simulink library "CaffeLibrary"  (Simulink 8.3)
settings: Solver=ode45  StartTime=0.0  StopTime=10.0  RelTol=1e-3
undefined symbols (not defined in the file): c_bias_term_, c_f_max_w, c_f_mean_w, c_f_min_w, c_f_std_w, c_f_type_b, c_f_type_w, c_f_value_w, c_f_variance_norm_w, c_group_, c_kernel_h_, c_kernel_w_, c_num_output_, c_stride_h_, c_stride_w_, EuclideanLoss, loss_weight, misc_, name_, Neuron, p_decay_b, p_decay_w, p_lr_b, p_lr_w, Pooling
settings Model: Creator=twerd  LastModifiedBy=gipadmin

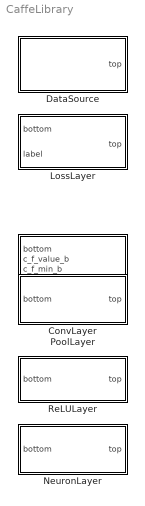
== system CaffeLibrary ==
  ConvLayer : MATLAB Function  TreatAsAtomicUnit=on  mask{title=0, numFilters=24.759999999999998, kernelSize=1.0, stride=0, weightFill=Xavier, weightStd=0, biasFill=0, biasVal=0}
      mask prompts: title "Name"; numFilters "Number of filters"; kernelSize "Kernel size"; weightFill "Type of weights"; weightStd "Std of weights"; biasFill "Type of biases"; biasVal "Bias value"
  DataSource : MATLAB Function  TreatAsAtomicUnit=on  mask{title=HDF5, srcFile=file.txt, batchSize=58}
      mask prompts: title "Name"; srcFile "Training files"; batchSize "Batch size"
  LossLayer : MATLAB Function  TreatAsAtomicUnit=on  mask{title=EuclideanLoss}
      mask prompts: title "Name"
  NeuronLayer : MATLAB Function  TreatAsAtomicUnit=on  mask{title=Neuron, typeOf=Sigmoid}
      mask prompts: title "Name"; typeOf "Type of neuron"
  PoolLayer : MATLAB Function  TreatAsAtomicUnit=on  mask{title=Pooling, poolType=MAX, kernelSize=1.000, stride=0.0}
      mask prompts: title "Name"; poolType "Type of pooling"; kernelSize "Size of kernel"
  ReLULayer : MATLAB Function  TreatAsAtomicUnit=on

== matlab function LossLayer ==
  data: title parameter int8; top output double; bottom input double; label input double
function top  = Euclidean(title, bottom, label)

coder.extrinsic('sprintf');
coder.extrinsic('fprintf');
coder.extrinsic('fopen');
coder.extrinsic('fclose');

str = sprintf( ...
 ['\nlayer {\n', ...
'  name: "%s"\n', ...
'  type: "EuclideanLoss"\n', ...
'  bottom: "%s"\n', ...
'  bottom: "%s"\n', ...
'  top: "loss"\n', ...
'}\n\n'], ...
 title, bottom, label);


f=fopen(char([title' '.txt']),'w');
fprintf(f,'%s',str);
fclose(f);

top = title;

== matlab function DataSource ==
  data: title parameter int8; srcFile parameter int8; top output double; batchSize parameter uint32
function top  = HDF5(title,srcFile,batchSize) 

coder.extrinsic('sprintf');
coder.extrinsic('fprintf');
coder.extrinsic('fopen');
coder.extrinsic('fclose');

dataName = 'data';
labelName = 'label';

str = sprintf( ...
 ['\nlayer {\n', ...
 ' name: "%s"\n',  ...
 ' type: "HDF5Data"\n', ...
 ' top: "%s"\n', ...
 ' top: "%s"\n', ...
 ' hdf5_data_param {\n', ...
 '   source: "%s"\n', ... %examples/hdf5_classification/data/train.txt
 '   batch_size: %i\n', ...
 ' }\n', ...
 '}\n\n'], ...
 title, dataName, labelName, srcFile, batchSize);


f=fopen(char([title' '.txt']),'w');
fprintf(f,'%s',str);
fclose(f);

top = title;

== matlab function ConvLayer ==
  data: name_ parameter double; bottom input double; top output double; loss_weight parameter uint32; misc_ parameter uint32; p_lr_w parameter uint32; p_decay_w parameter int8; p_lr_b parameter single; p_decay_b parameter int8; c_group_ parameter single; c_bias_term_ parameter double; c_num_output_ parameter double; c_kernel_w_ parameter double; c_kernel_h_ parameter double; c_stride_w_ parameter double; c_stride_h_ parameter double; c_f_type_w parameter double; c_f_value_w parameter double; c_f_min_w parameter double; c_f_max_w parameter double; c_f_mean_w parameter double; c_f_std_w parameter double; c_f_variance_norm_w parameter double; c_f_type_b parameter double; c_f_value_b input double; c_f_min_b input double; c_f_max_b input double; c_f_mean_b input double; c_f_std_b input double; c_f_variance_norm_b input double
function top  =  Convolution(name_, bottom,loss_weight, misc_, ...
p_lr_w, p_decay_w, p_lr_b, p_decay_b, ...
c_group_,c_bias_term_,c_num_output_,c_kernel_w_,c_kernel_h_,c_stride_w_,c_stride_h_, ...
c_f_type_w,c_f_value_w,c_f_min_w,c_f_max_w,c_f_mean_w,c_f_std_w,c_f_variance_norm_w, ...
c_f_type_b,c_f_value_b,c_f_min_b,c_f_max_b,c_f_mean_b,c_f_std_b,c_f_variance_norm_b)


coder.extrinsic('sprintf');
coder.extrinsic('fprintf');
coder.extrinsic('fopen');
coder.extrinsic('fclose');

s = @(x,fmt) sprintf(fmt,x);

str = [ ...
'\nlayer {\n', ...
'  name: "' s(name_ , '%s')  '"\n', ...
'  type: "Convolution"\n', ...
'  bottom: "' s(bottom , '%s')  '"\n', ...
'  top: "' s(name_ , '%s')  '"\n', ...
'  loss_weight: ' s(loss_weight , '%.1f')  '\n', ...
   s(misc_ , '%s'), ... % additional layer parameters entered by user
'  param { lr_mult: ' s(p_lr_w , '%i')  ' decay_mult: ' s(p_decay_w , '%i')  ' }  # learning rate and decay multipliers for the filters\n', ...
'  param { lr_mult: ' s(p_lr_b , '%i')  ' decay_mult: ' s(p_decay_b , '%i')  ' } # learning rate and decay multipliers for the biases\n', ...
'  convolution_param {\n', ...
'    group: ' s(c_group_ , '%i')  '          # The group size for group conv\n', ...
'    bias_term: ' s(c_bias_term_ , '%s')  '      # whether to use bias terms(true,false)\n', ...
'    num_output: ' s(c_num_output_ , '%i')  '     # The number of outputs for the layer\n', ...
'    kernel_w: ' s(c_kernel_w_ , '%i')  '       # The kernel width\n', ...
'    kernel_h: ' s(c_kernel_h_ , '%i')  '       # The kernel height\n', ...
'    stride_w: ' s(c_stride_w_ , '%i')  '       # The stride width\n', ...
'    stride_h: ' s(c_stride_h_ , '%i')  '       # The stride height\n', ...
'    weight_filler {\n', ...
'      type: "' s(c_f_type_w , '%s')  '"       # Filler type\n', ...
'      value: ' s(c_f_value_w , '%f')  ' # the value in constant filler\n', ...
'      min: ' s(c_f_min_w , '%f')  ' # the min value in uniform filler\n', ...
'      max: ' s(c_f_max_w , '%f')  ' # the max value in uniform filler\n', ...
'      mean: ' s(c_f_mean_w , '%f')  ' # the mean value in Gaussian filler\n', ...
'      std: ' s(c_f_std_w , '%f')  ' # the std value in Gaussian filler\n', ...
'      variance_norm: ' s(c_f_variance_norm_w , '%s')  ' # Normalize the filler variance by fan_in, fan_out, or their average.\n', ...
'    }\n', ...  
'    bias_filler {\n', ...
'      type: "' s(c_f_type_b , '%s' )  '"       # Filler type\n', ...
'      value: ' s(c_f_value_b , '%f')  ' # the value in constant filler\n', ...
'      min: ' s(c_f_min_b , '%f')  ' # the min value in uniform filler\n', ...
'      max: ' s(c_f_max_b , '%f')  ' # the max value in uniform filler\n', ...
'      mean:' s(c_f_mean_b , '%f')  ' # the mean value in Gaussian filler\n', ...
'      std: ' s(c_f_std_b , '%f')  ' # the std value in Gaussian filler\n', ...
'      variance_norm: ' s(c_f_variance_norm_b , '%s')  ' # Normalize the filler variance by fan_in, fan_out, or their average.\n', ...
'    }\n', ...  
'  }\n', ...
'}\n\n'];

f=fopen(char([title' '.txt']),'w');
fprintf(f,'%s',str);
fclose(f);

top = title; 



% 
%   Phase_ENUM = {'TRAIN','TEST'}; Use this for data layers only
%   Engine_ENUM = {'DEFAULT','CAFFE','CUDNN'}; 
%   Filler_ENUM = {'constant','gaussian','positive_unitball','uniform','xavier','msra','bilinear'};
%   Variance_Norm_ENUM = {'FAN_IN','FAN_OUT','AVERGAE'};
%   
%   name = 1; # the layer name
%   type = 2; # the layer type
%   bottom = 3; # the name of each bottom blob
%   top = 4; # the name of each top blob
%   phase = 10; # The train / test phase for computation.
%   loss_weight = 5;# The amount of weight to assign each top blob in the objective. Each layer assigns a default value, usually of either 0 or 1, to each top blob.
%   repeated ParamSpec param = 6;  # Specifies training parameters (multipliers on global learning constants,and the name and other settings used for weight sharing).
% 
%   
%   constant: value,sparse
%   uniform: min,max,sparse
%   gaussian: mean,std,sparse
%   positiveunitball:sparse
%   xavier:variance_norm,sparse
%   msra:variance_norm,sparse
%   bilinear: sparse
% 
%  (...  
% '    weight_filler {\n', ...
% '      type: "%s"       # Filler type\n', ...
% '      value: %f # the value in constant filler\n', ...
% '      min: %f # the min value in uniform filler\n', ...
% '      max: %f # the max value in uniform filler\n', ...
% '      mean: %f # the mean value in Gaussian filler\n', ...
% '      std: %f # the std value in Gaussian filler\n', ...
% '      sparse: %i\n', ...
% '      VarianceNorm: %s # Normalize the filler variance by fan_in, fan_out, or their average.\n', ...
% '    }\n', ...  
% '    bias_filler {\n', ...
% '      type: "%s"       # Filler type\n', ...
% '      value: %f # the value in constant filler\n', ...
% '      min: %f # the min value in uniform filler\n', ...
% '      max: %f # the max value in uniform filler\n', ...
% '      mean: %f # the mean value in Gaussian filler\n', ...
% '      std: %f # the std value in Gaussian filler\n', ...
% '      sparse: %i\n', ...
% '      VarianceNorm: %s # Normalize the filler variance by fan_in, fan_out, or their average.\n', ...
% '    }\n', ...  
% 
%   );

== matlab function PoolLayer ==
  data: title parameter int8; top output double; bottom input double; poolType parameter double; kernelSize parameter double; stride parameter double
function top  = Pooling(title, bottom, poolType, kernelSize,stride)

coder.extrinsic('sprintf');
coder.extrinsic('fprintf');
coder.extrinsic('fopen');
coder.extrinsic('fclose');

str = sprintf( ...
'layer {\n', ...
'  name: "%s"\n', ...
'  type: "Pooling"\n', ...
'  bottom: "%s"\n', ...
'  top: "%s"\n', ...
'  pooling_param {\n', ...
'    pool: %s\n', ...
'    kernel_size: %i # pool over a %iX%i region\n', ...
'    stride: %i      # step %i pixels (in the bottom blob) between pooling regions\n', ...
'  }\n', ...
'}\n', ...
title, bottom, title, poolType, kernelSize,kernelSize,kernelSize, stride,stride );

f=fopen(char([title' '.txt']),'w');
fprintf(f,'%s',str);
fclose(f);

top = title;

== matlab function ReLULayer ==
  data: bottom input double; top output double
function top  = ReLU(bottom)

coder.extrinsic('sprintf');
coder.extrinsic('fprintf');
coder.extrinsic('fopen');
coder.extrinsic('fclose');

str = sprintf( ...
'layer {\n', ...
'  name: "%s"\n', ...
'  type: "ReLU"\n', ...
'  bottom: "%s"\n', ...
'  top: "%s"\n', ...
'}\n', ...
bottom, bottom, bottom);

f=fopen(char([bottom' '.txt']),'w');
fprintf(f,'%s',str);
fclose(f);

top = bottom;

== matlab function NeuronLayer ==
  data: title parameter uint8; top output double; bottom input double; typeOf parameter int8
function top  = Neuron(title, bottom, typeOf)

coder.extrinsic('sprintf');
coder.extrinsic('fprintf');
coder.extrinsic('fopen');
coder.extrinsic('fclose');

str = sprintf( ...
'layer {\n', ...
'  name: "%s"\n', ...
'  bottom: "%s"\n', ...
'  top: "%s"\n', ...
'  type: "%s"\n', ...
'}\n', ...
title, bottom, title, typeOf);

f=fopen(char([title' '.txt']),'w');
fprintf(f,'%s',str);
fclose(f);

top = title;
